simulink model "r_pendulo"  (R2024b)
settings: Solver=ode45  StartTime=0.0  StopTime=10.0  RelTol=1e-3
InitFcn:
  | g = 9.81;
  | Mc = 0.7031;
  | Mp = 0.23;
  | Ip = 0.0079;
  | lp = 0.3302;
  | Beq = 4.3;
  | Bp = 0.0024;
model workspace (MAT data in the model file):
  Beq = 4.3
  Bp = 0.0024
  Fc = 0
  Ip = 0.0079
  Lp = 0.3302
  Mc = 0.7031
  Mp = 0.23
  a = 0.0174533
  g = 9.81
settings Model: Creator=DELL  LastModifiedBy=DELL

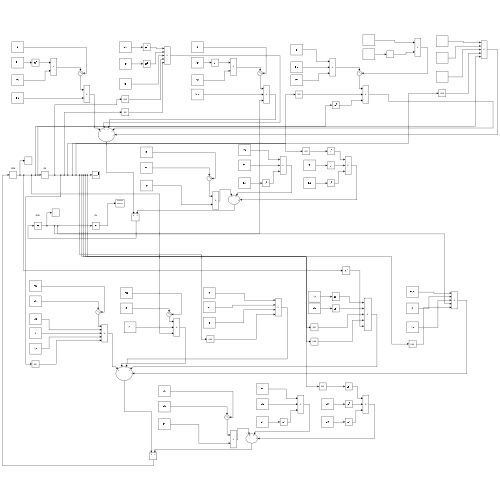
[thumbnail: Simulink's stored preview of the top-level diagram]
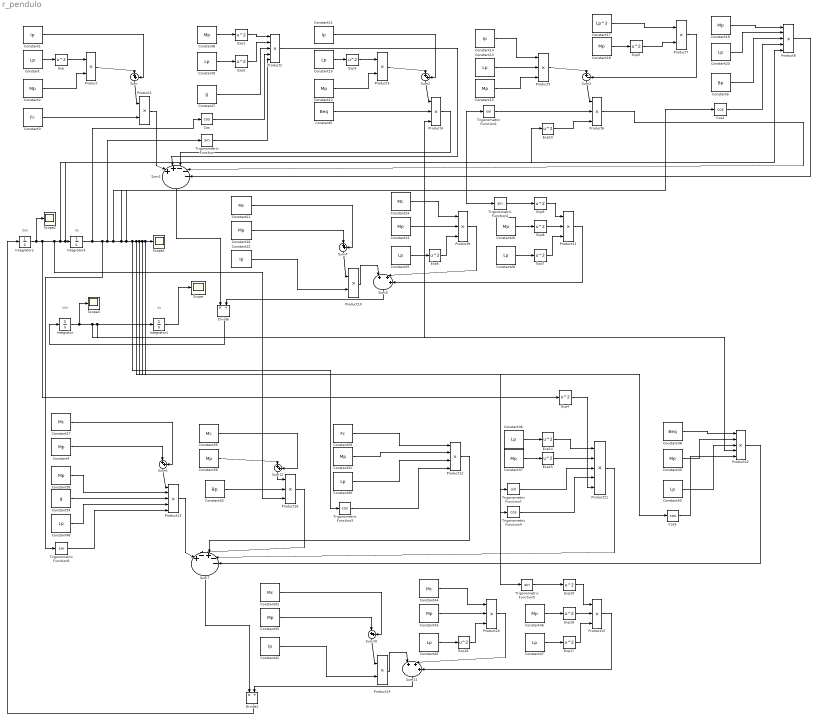
== system r_pendulo ==
  note: dx
  note: ddx
  note: da
  note: dda
  Constant{,9..10,13,20,25,28,30,36,45,47..48,50} (13 alike) : Constant  Value=Lp
  Constant{1,11,14,22,42} (5 alike) : Constant  Value=Ip
  Constant{2,4,8,12,15..16,18..19,23,26,31,35,37,39..40,43,46,56} (18 alike) : Constant  Value=Mp
  Constant17 : Constant  Value=Lp^3
  Constant{21,24,27,41,44,55} (6 alike) : Constant  Value=Mc
  Constant29 : Constant  Value=Fc
  Constant3 : Constant  Value=Fc
  Constant38 : Constant  Value=Beq
  Constant5 : Constant  Value=Beq
  Constant52 : Constant  Value=Bp
  Constant54 : Constant  Value=g
  Constant6 : Constant  Value=Bp
  Constant7 : Constant  Value=g
  Cos : Trigonometry  Operator=cos
  Cos1 : Trigonometry  Operator=cos
  Cos3 : Trigonometry  Operator=cos
  Divide : Product  Inputs=*/
  Divide1 : Product  Inputs=*/
  Exp{,1..10,14..19} (17 alike) : Math  Operator=square
  Integrator : Integrator
  Integrator1 : Integrator
  Integrator2 : Integrator
  Integrator3 : Integrator  InitialCondition=0.0174533
  Product{,1,3,7,10,14} (6 alike) : Product
  Product{4..6,9,11,15..16,23} (8 alike) : Product  Inputs=3
  Product12 : Product  Inputs=4
  Product{2,8,13,21..22} (5 alike) : Product  Inputs=5
  Scope{,1..3} (4 alike) : Scope
  Sum{,2,4,6,10,12} (6 alike) : Sum  Inputs=|++
  Sum1 : Sum  Inputs=|++---
  Sum11 : Sum  Inputs=|+++
  Sum3 : Sum  Inputs=|+-
  Sum5 : Sum  Inputs=|+++
  Sum7 : Sum  Inputs=|+-+--
  Trigonometric Function{,1..2,5..7} (6 alike) : Trigonometry
  Trigonometric Function3 : Trigonometry  Operator=cos
  Trigonometric Function4 : Trigonometry  Operator=cos
  wires:
  Constant/1 -> Exp/1
  Exp/1 -> Product/1
  Constant2/1 -> Product/2
  Product/1 -> Sum/1
  Constant1/1 -> Sum/2
  Sum/1 -> Product1/1
  Constant3/1 -> Product1/2
  Product1/1 -> Sum1/1
  Constant8/1 -> Exp1/1
  Constant9/1 -> Exp2/1
  Exp1/1 -> Product2/1
  Exp2/1 -> Product2/2
  Constant7/1 -> Product2/3
  Cos/1 -> Product2/4
  Trigonometric Function/1 -> Product2/5
  Product2/1 -> Sum1/2
  Constant5/1 -> Product4/2
  Constant12/1 -> Product3/2
  Sum2/1 -> Product4/1
  Constant11/1 -> Sum2/2
  Product3/1 -> Sum2/1
  Constant10/1 -> Exp3/1
  Exp3/1 -> Product3/1
  Product4/1 -> Sum1/3
  Product5/1 -> Sum3/1
  Product6/1 -> Sum1/4
  Constant15/1 -> Product5/3
  Sum3/1 -> Product6/1
  Trigonometric Function1/1 -> Product6/2
  Constant13/1 -> Product5/2
  Constant14/1 -> Product5/1
  Constant17/1 -> Product7/1
  Constant18/1 -> Exp5/1
  Exp5/1 -> Product7/2
  Product7/1 -> Sum3/2
  Product8/1 -> Sum1/5
  Cos1/1 -> Product8/4
  Constant19/1 -> Product8/1
  Constant20/1 -> Product8/2
  Constant6/1 -> Product8/3
  Sum4/1 -> Product10/1
  Constant21/1 -> Sum4/2
  Constant16/1 -> Sum4/1
  Constant22/1 -> Product10/2
  Product10/1 -> Sum5/1
  Constant24/1 -> Product9/1
  Constant23/1 -> Product9/2
  Constant25/1 -> Exp6/1
  Exp6/1 -> Product9/3
  Product9/1 -> Sum5/2
  Exp7/1 -> Product11/3
  Constant28/1 -> Exp7/1
  Product11/1 -> Sum5/3
  Constant26/1 -> Exp8/1
  Exp8/1 -> Product11/2
  Sum1/1 -> Divide/1
  Sum5/1 -> Divide/2
  Divide/1 -> Integrator/1
  Integrator1/1 -> Scope/1
  Constant40/1 -> Product22/2
  Exp15/1 -> Product21/2
  Sum7/1 -> Divide1/1
  Exp16/1 -> Product23/3
  Integrator3/1 -> Cos/1, Trigonometric Function6/1, Trigonometric Function/1, Trigonometric Function1/1, Cos1/1, Trigonometric Function2/1, Trigonometric Function3/1, Trigonometric Function7/1, Trigonometric Function4/1, Cos3/1, Trigonometric Function5/1, Scope1/1
  Constant46/1 -> Exp18/1
  Constant36/1 -> Exp14/1
  Product12/1 -> Sum7/3
  Divide1/1 -> Integrator2/1
  Constant44/1 -> Product23/1
  Product23/1 -> Sum11/2
  Product16/1 -> Sum7/2
  Constant42/1 -> Product14/2
  Constant35/1 -> Sum10/1
  Product13/1 -> Sum7/1
  Constant50/1 -> Product22/3
  Constant41/1 -> Sum10/2
  Product21/1 -> Sum7/4
  Exp18/1 -> Product15/2
  Constant48/1 -> Product13/4
  Constant27/1 -> Sum6/2
  Constant38/1 -> Product22/1
  Sum10/1 -> Product14/1
  Cos3/1 -> Product22/5
  Constant45/1 -> Exp16/1
  Sum6/1 -> Product13/1
  Constant37/1 -> Exp15/1
  Sum11/1 -> Divide1/2
  Constant47/1 -> Exp17/1
  Product14/1 -> Sum11/1
  Exp17/1 -> Product15/3
  Product22/1 -> Sum7/5
  Constant43/1 -> Product23/2
  Exp14/1 -> Product21/1
  Product15/1 -> Sum11/3
  Constant4/1 -> Sum6/1
  Constant39/1 -> Product13/2
  Constant54/1 -> Product13/3
  Trigonometric Function6/1 -> Product13/5
  Constant56/1 -> Sum12/1
  Constant55/1 -> Sum12/2
  Constant52/1 -> Product16/2
  Sum12/1 -> Product16/1
  Constant29/1 -> Product12/1
  Constant30/1 -> Product12/3
  Constant31/1 -> Product12/2
  Trigonometric Function3/1 -> Product12/4
  Trigonometric Function7/1 -> Product21/3
  Trigonometric Function4/1 -> Product21/4
  Integrator/1 -> Product22/4, Product4/3, Integrator1/1, Scope3/1
  Integrator2/1 -> Scope2/1, Exp4/1, Product16/3, Exp10/1, Integrator3/1, Product8/5
  Exp4/1 -> Product21/5
  Exp10/1 -> Product6/3
  Trigonometric Function2/1 -> Exp9/1
  Exp9/1 -> Product11/1
  Trigonometric Function5/1 -> Exp19/1
  Exp19/1 -> Product15/1
